simulink model "BLDC_Speed_Torque_Current_ClosedLoop"  (R2022b)
settings: Solver=ode4  StartTime=0.0  StopTime=3  FixedStep=1e-6  RelTol=1e-3
model workspace (MAT data in the model file):
  Ctrol_Mode = 4
  Current_Control_Mode = 2
  Current_PID_Upper_Limit = 1
  PWM_Period = 0.0001
  Speed_I = 10
  Speed_P = 10
  Speed_PID_Upper_Limit = 0.02
  Ts_time = 1e-06
  current_I = 10
  current_P = 100
undefined symbols (not defined in the file): DiscIntNeverNeededParam, sigbuilder_block
libraries: simulink x18, slpidlib x6, dsparch4 x3, eePwmGenerator x3, spsSeriesRLCBranchLib x2, spsPermanentMagnetSynchronousMachineLib x1, spsCurrentMeasurementLib x1, spsDCVoltageSourceLib x1, slctrlblks x1, spsTwoLevelConverterLib x1, spspowerguiLib x1
(part 2 of 2)

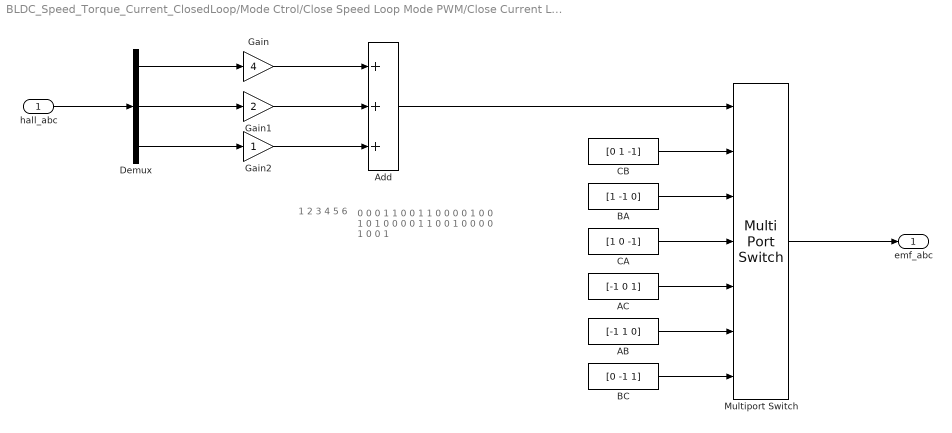
== system BLDC_Speed_Torque_Current_ClosedLoop/Mode Ctrol/Close Speed Loop Mode PWM/Close Current Loop Mode PWM/反转逻辑 ==
  note: 0 0 0 1 1 0
      | 0 1 1 0 0 0
      | 0 1 0 0 1 0
      | 1 0 0 0 0 1
      | 1 0 0 1 0 0
      | 0 0 1 0 0 1
  note: 1
      | 2
      | 3
      | 4
      | 5
      | 6
  hall_abc : Inport
  AB : Constant  Value=[-1 1 0]
  AC : Constant  Value=[-1 0 1]
  Add : Sum  Inputs=+++
  BA : Constant  Value=[1 -1 0]
  BC : Constant  Value=[0 -1 1]
  CA : Constant  Value=[1 0 -1]
  CB : Constant  Value=[0 1 -1]
  Demux : Demux  Outputs=3
  Gain : Gain  Gain=4
  Gain1 : Gain  Gain=2
  Gain2 : Gain
  Multiport Switch : MultiPortSwitch  Inputs=6  DiagnosticForDefault=None  SaturateOnIntegerOverflow=off  InputSameDT=off
  emf_abc : Outport
  wires:
  BA/1 -> Multiport Switch/3
  CB/1 -> Multiport Switch/2
  CA/1 -> Multiport Switch/4
  AB/1 -> Multiport Switch/6
  BC/1 -> Multiport Switch/7
  Multiport Switch/1 -> emf_abc/1
  Add/1 -> Multiport Switch/1
  AC/1 -> Multiport Switch/5
  Gain/1 -> Add/1
  Gain1/1 -> Add/2
  Gain2/1 -> Add/3
  Demux/2 -> Gain1/1
  Demux/1 -> Gain/1
  Demux/3 -> Gain2/1
  hall_abc/1 -> Demux/1

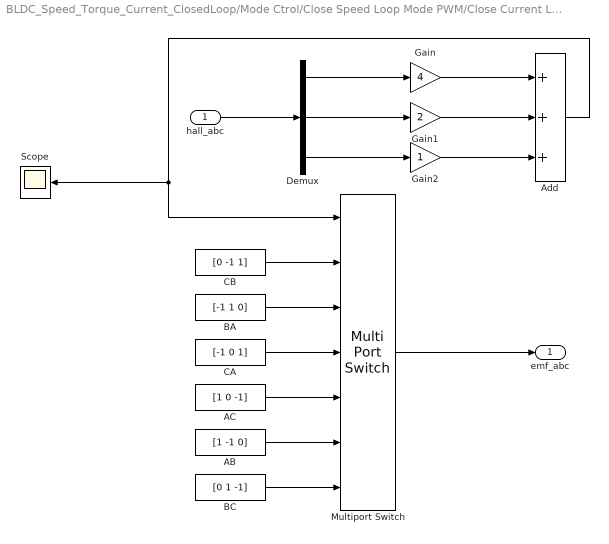
== system BLDC_Speed_Torque_Current_ClosedLoop/Mode Ctrol/Close Speed Loop Mode PWM/Close Current Loop Mode PWM/正转逻辑 ==
  hall_abc : Inport
  AB : Constant  Value=[1 -1 0]
  AC : Constant  Value=[1 0 -1]
  Add : Sum  Inputs=+++
  BA : Constant  Value=[-1 1 0]
  BC : Constant  Value=[0 1 -1]
  CA : Constant  Value=[-1 0 1]
  CB : Constant  Value=[0 -1 1]
  Demux : Demux  Outputs=3
  Gain : Gain  Gain=4
  Gain1 : Gain  Gain=2
  Gain2 : Gain
  Multiport Switch : MultiPortSwitch  Inputs=6  DiagnosticForDefault=None  SaturateOnIntegerOverflow=off  InputSameDT=off
  Scope : Scope
  emf_abc : Outport
  wires:
  BA/1 -> Multiport Switch/3
  CB/1 -> Multiport Switch/2
  CA/1 -> Multiport Switch/4
  AB/1 -> Multiport Switch/6
  BC/1 -> Multiport Switch/7
  Multiport Switch/1 -> emf_abc/1
  Add/1 -> Scope/1, Multiport Switch/1
  AC/1 -> Multiport Switch/5
  Gain/1 -> Add/1
  Gain1/1 -> Add/2
  Gain2/1 -> Add/3
  Demux/2 -> Gain1/1
  Demux/1 -> Gain/1
  Demux/3 -> Gain2/1
  hall_abc/1 -> Demux/1

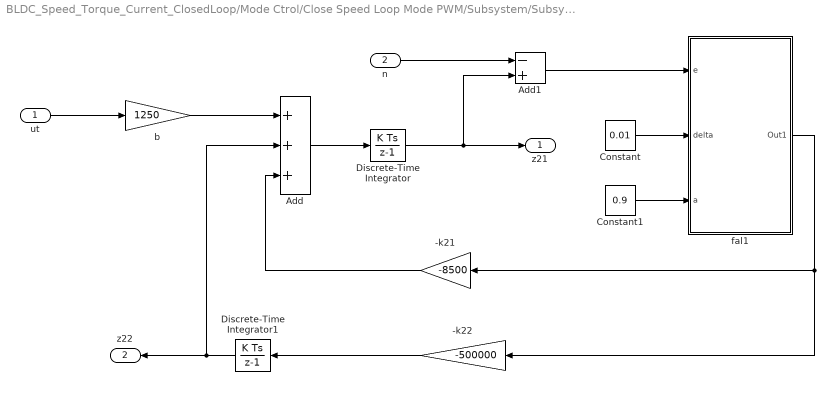
== system BLDC_Speed_Torque_Current_ClosedLoop/Mode Ctrol/Close Speed Loop Mode PWM/Subsystem/Subsystem2 ==
  ut : Inport
  n : Inport  Port=2
  -k21 : Gain  Gain=-8500
  -k22 : Gain  Gain=-500000
  Add : Sum  Inputs=+++
  Add1 : Sum  Inputs=-+
  Constant : Constant  Value=0.01
  Constant1 : Constant  Value=0.9
  Discrete-Time Integrator : DiscreteIntegrator  SampleTime=-1  ICPrevOutput=DiscIntNeverNeededParam  ICPrevScaledInput=DiscIntNeverNeededParam
  Discrete-Time Integrator1 : DiscreteIntegrator  SampleTime=-1  ICPrevOutput=DiscIntNeverNeededParam  ICPrevScaledInput=DiscIntNeverNeededParam
  b : Gain  Gain=1250
  fal1 : Subsystem
  z21 : Outport
  z22 : Outport  Port=2
  wires:
  ut/1 -> b/1
  b/1 -> Add/1
  Add/1 -> Discrete-Time Integrator/1
  n/1 -> Add1/1
  Discrete-Time Integrator/1 -> z21/1, Add1/2
  Add1/1 -> fal1/1(e)
  fal1/1(Out1) -> -k21/1, -k22/1
  -k22/1 -> Discrete-Time Integrator1/1
  -k21/1 -> Add/3
  Discrete-Time Integrator1/1 -> z22/1, Add/2
  Constant/1 -> fal1/2(delta)
  Constant1/1 -> fal1/3(a)

== system BLDC_Speed_Torque_Current_ClosedLoop/Mode Ctrol/Close Speed Loop Mode PWM/Subsystem/TD ==
  n* : Inport
  -k0 : Gain  Gain=-6500
  Add : Sum  Inputs=-+
  Discrete-Time Integrator : DiscreteIntegrator  SampleTime=-1  ICPrevOutput=DiscIntNeverNeededParam  ICPrevScaledInput=DiscIntNeverNeededParam
  Scope : Scope
  a0 : Constant  Value=0.4
  delta0 : Constant  Value=0.01
  fal : Subsystem
  z11 : Outport
  wires:
  n*/1 -> Add/1
  Discrete-Time Integrator/1 -> Add/2, z11/1
  fal/1(Out1) -> Scope/1, -k0/1
  -k0/1 -> Discrete-Time Integrator/1
  Add/1 -> fal/1(e)
  delta0/1 -> fal/2(delta)
  a0/1 -> fal/3(a)

== system BLDC_Speed_Torque_Current_ClosedLoop/Mode Ctrol/Close Speed Loop Mode PWM/Subsystem/nlsef ==
  z11 : Inport
  z22 : Inport  Port=2
  z21 : Inport  Port=3
  1/b : Gain  Gain=1/1000
  Add : Sum  Inputs=+-
  Add1 : Sum  Inputs=-+
  Constant : Constant  Value=0.01
  Constant1 : Constant  Value=0.9
  Scope : Scope
  fal1 : Subsystem
  k3 : Gain  Gain=5000
  ut : Outport
  wires:
  z11/1 -> Add/1
  z21/1 -> Add/2
  z22/1 -> 1/b/1
  Add1/1 -> ut/1
  k3/1 -> Add1/2
  fal1/1(Out1) -> Scope/1, k3/1  "u0"
  1/b/1 -> Add1/1
  Add/1 -> fal1/1(e)
  Constant/1 -> fal1/2(delta)
  Constant1/1 -> fal1/3(a)

== system BLDC_Speed_Torque_Current_ClosedLoop/Mode Ctrol/Close Speed Loop Mode PWM/一阶LADRC/ESO ==
  ut : Inport
  n : Inport  Port=2
  -k1=2w0 : Gain  Gain=-10
  -k2=w0^2 : Gain  Gain=-25
  Add : Sum  Inputs=+++
  Add1 : Sum  Inputs=-+
  Discrete-Time Integrator : DiscreteIntegrator  SampleTime=-1  ICPrevOutput=DiscIntNeverNeededParam  ICPrevScaledInput=DiscIntNeverNeededParam
  Discrete-Time Integrator1 : DiscreteIntegrator  SampleTime=-1  ICPrevOutput=DiscIntNeverNeededParam  ICPrevScaledInput=DiscIntNeverNeededParam
  z1 : Outport
  z2 : Outport  Port=2
  wires:
  Discrete-Time Integrator1/1 -> z2/1, Add/2
  -k2=w0^2/1 -> Discrete-Time Integrator1/1
  Add/1 -> Discrete-Time Integrator/1
  n/1 -> Add1/1
  -k1=2w0/1 -> Add/3
  Add1/1 -> -k2=w0^2/1, -k1=2w0/1  "e1"
  Discrete-Time Integrator/1 -> z1/1, Add1/2
  ut/1 -> Add/1

== system BLDC_Speed_Torque_Current_ClosedLoop/Mode Ctrol/Close Torque Loop Mode PWM/Close Current Loop Mode PWM/反转逻辑 ==
  note: 0 0 0 1 1 0
      | 0 1 1 0 0 0
      | 0 1 0 0 1 0
      | 1 0 0 0 0 1
      | 1 0 0 1 0 0
      | 0 0 1 0 0 1
  note: 1
      | 2
      | 3
      | 4
      | 5
      | 6
  hall_abc : Inport
  AB : Constant  Value=[-1 1 0]
  AC : Constant  Value=[-1 0 1]
  Add : Sum  Inputs=+++
  BA : Constant  Value=[1 -1 0]
  BC : Constant  Value=[0 -1 1]
  CA : Constant  Value=[1 0 -1]
  CB : Constant  Value=[0 1 -1]
  Demux : Demux  Outputs=3
  Gain : Gain  Gain=4
  Gain1 : Gain  Gain=2
  Gain2 : Gain
  Multiport Switch : MultiPortSwitch  Inputs=6  DiagnosticForDefault=None  SaturateOnIntegerOverflow=off  InputSameDT=off
  emf_abc : Outport
  wires:
  BA/1 -> Multiport Switch/3
  CB/1 -> Multiport Switch/2
  CA/1 -> Multiport Switch/4
  AB/1 -> Multiport Switch/6
  BC/1 -> Multiport Switch/7
  Multiport Switch/1 -> emf_abc/1
  Add/1 -> Multiport Switch/1
  AC/1 -> Multiport Switch/5
  Gain/1 -> Add/1
  Gain1/1 -> Add/2
  Gain2/1 -> Add/3
  Demux/2 -> Gain1/1
  Demux/1 -> Gain/1
  Demux/3 -> Gain2/1
  hall_abc/1 -> Demux/1

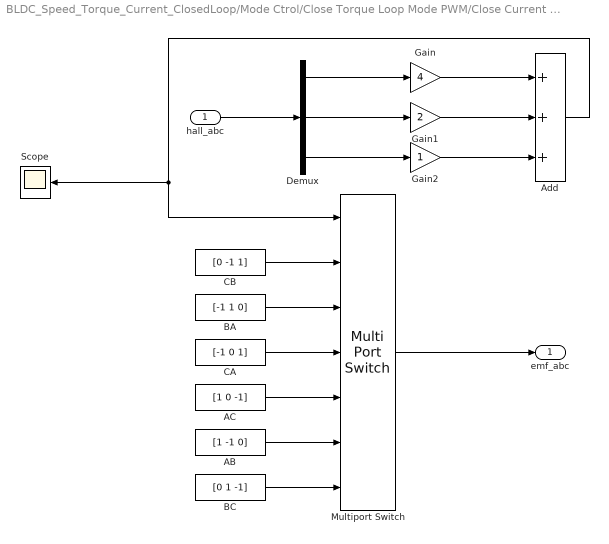
== system BLDC_Speed_Torque_Current_ClosedLoop/Mode Ctrol/Close Torque Loop Mode PWM/Close Current Loop Mode PWM/正转逻辑 ==
  hall_abc : Inport
  AB : Constant  Value=[1 -1 0]
  AC : Constant  Value=[1 0 -1]
  Add : Sum  Inputs=+++
  BA : Constant  Value=[-1 1 0]
  BC : Constant  Value=[0 1 -1]
  CA : Constant  Value=[-1 0 1]
  CB : Constant  Value=[0 -1 1]
  Demux : Demux  Outputs=3
  Gain : Gain  Gain=4
  Gain1 : Gain  Gain=2
  Gain2 : Gain
  Multiport Switch : MultiPortSwitch  Inputs=6  DiagnosticForDefault=None  SaturateOnIntegerOverflow=off  InputSameDT=off
  Scope : Scope
  emf_abc : Outport
  wires:
  BA/1 -> Multiport Switch/3
  CB/1 -> Multiport Switch/2
  CA/1 -> Multiport Switch/4
  AB/1 -> Multiport Switch/6
  BC/1 -> Multiport Switch/7
  Multiport Switch/1 -> emf_abc/1
  Add/1 -> Scope/1, Multiport Switch/1
  AC/1 -> Multiport Switch/5
  Gain/1 -> Add/1
  Gain1/1 -> Add/2
  Gain2/1 -> Add/3
  Demux/2 -> Gain1/1
  Demux/1 -> Gain/1
  Demux/3 -> Gain2/1
  hall_abc/1 -> Demux/1

== system BLDC_Speed_Torque_Current_ClosedLoop/Mode Ctrol/Close Speed Loop Mode PWM/Subsystem/Subsystem2/fal1 ==
  e : Inport
  delta : Inport  Port=2
  a : Inport  Port=3
  Abs : Abs  SaturateOnIntegerOverflow=off
  Add : Sum  Inputs=+-
  Add1 : Sum  Inputs=-+
  Constant : Constant
  Divide : Product  Inputs=*/
  Math Function : Math  Operator=pow  SignedPower=on
  Math Function1 : Math  Operator=pow  SignedPower=on
  Product : Product
  Sign : Signum
  Switch : Switch  Criteria=u2 > Threshold  SaturateOnIntegerOverflow=off  InputSameDT=off
  Out1 : Outport
  wires:
  e/1 -> Abs/1, Divide/1, Sign/1
  Sign/1 -> Product/1
  delta/1 -> Math Function1/1, Add/2
  Abs/1 -> Add/1, Math Function/1
  Add/1 -> Switch/2
  Product/1 -> Switch/1
  Divide/1 -> Switch/3
  a/1 -> Math Function/2, Add1/1
  Constant/1 -> Add1/2
  Add1/1 -> Math Function1/2
  Math Function1/1 -> Divide/2
  Math Function/1 -> Product/2
  Switch/1 -> Out1/1

== system BLDC_Speed_Torque_Current_ClosedLoop/Mode Ctrol/Close Speed Loop Mode PWM/Subsystem/TD/fal ==
  e : Inport
  delta : Inport  Port=2
  a : Inport  Port=3
  Abs : Abs  SaturateOnIntegerOverflow=off
  Add : Sum  Inputs=+-
  Add1 : Sum  Inputs=-+
  Constant : Constant
  Divide : Product  Inputs=*/
  Math Function : Math  Operator=pow  SignedPower=on
  Math Function1 : Math  Operator=pow  SignedPower=on
  Product : Product
  Sign : Signum
  Switch : Switch  Criteria=u2 > Threshold  SaturateOnIntegerOverflow=off  InputSameDT=off
  Out1 : Outport
  wires:
  e/1 -> Abs/1, Divide/1, Sign/1
  Sign/1 -> Product/1
  delta/1 -> Math Function1/1, Add/2
  Abs/1 -> Add/1, Math Function/1
  Add/1 -> Switch/2
  Product/1 -> Switch/1
  Divide/1 -> Switch/3
  a/1 -> Math Function/2, Add1/1
  Constant/1 -> Add1/2
  Add1/1 -> Math Function1/2
  Math Function1/1 -> Divide/2
  Math Function/1 -> Product/2
  Switch/1 -> Out1/1

== system BLDC_Speed_Torque_Current_ClosedLoop/Mode Ctrol/Close Speed Loop Mode PWM/Subsystem/nlsef/fal1 ==
  e : Inport
  delta : Inport  Port=2
  a : Inport  Port=3
  Abs : Abs  SaturateOnIntegerOverflow=off
  Add : Sum  Inputs=+-
  Add1 : Sum  Inputs=-+
  Constant : Constant
  Divide : Product  Inputs=*/
  Math Function : Math  Operator=pow  SignedPower=on
  Math Function1 : Math  Operator=pow  SignedPower=on
  Product : Product
  Sign : Signum
  Switch : Switch  Criteria=u2 > Threshold  SaturateOnIntegerOverflow=off  InputSameDT=off
  Out1 : Outport
  wires:
  e/1 -> Abs/1, Divide/1, Sign/1
  Sign/1 -> Product/1
  delta/1 -> Math Function1/1, Add/2
  Abs/1 -> Add/1, Math Function/1
  Add/1 -> Switch/2
  Product/1 -> Switch/1
  Divide/1 -> Switch/3
  a/1 -> Math Function/2, Add1/1
  Constant/1 -> Add1/2
  Add1/1 -> Math Function1/2
  Math Function1/1 -> Divide/2
  Math Function/1 -> Product/2
  Switch/1 -> Out1/1

== matlab function BLDC_Speed_Torque_Current_ClosedLoop/MATLAB Function2 ==
  data: angle input; theta output
function theta = Angle_Conv(angle)

n=mod(angle,pi);

theta = n;

== matlab function BLDC_Speed_Torque_Current_ClosedLoop/MATLAB Function1 ==
  data: Hall_a input; sign_a output; Hall_b input; Hall_c input; sign_b output; sign_c output
function [sign_a,sign_b,sign_c] = fcn(Hall_a, Hall_b, Hall_c)

if Hall_a==1&&Hall_b==0&&Hall_c==1

sign_a=1;
sign_b=0;
sign_c=-1;

elseif Hall_a==1&&Hall_b==0&&Hall_c==0

sign_a=0;
sign_b=1;
sign_c=-1;


elseif Hall_a==1&&Hall_b==1&&Hall_c==0

sign_a=-1;
sign_b=1;
sign_c=0;


elseif Hall_a==0&&Hall_b==1&&Hall_c==0

sign_a=-1;
sign_b=0;
sign_c=1;


elseif Hall_a==0&&Hall_b==1&&Hall_c==1

sign_a=0;
sign_b=-1;
sign_c=1;

else

sign_a=1;
sign_b=-1;
sign_c=0;


end
